simulink model "WiperSystem"  (R2016a)
settings: Solver=FixedStepDiscrete  StartTime=0.0  StopTime=20  FixedStep=0.01  RelTol=1e-3
undefined symbols (not defined in the file): sigbuilder_block
libraries: simulink x1
settings Model: Creator=Kimo Store  LastModifiedBy=Kimo Store

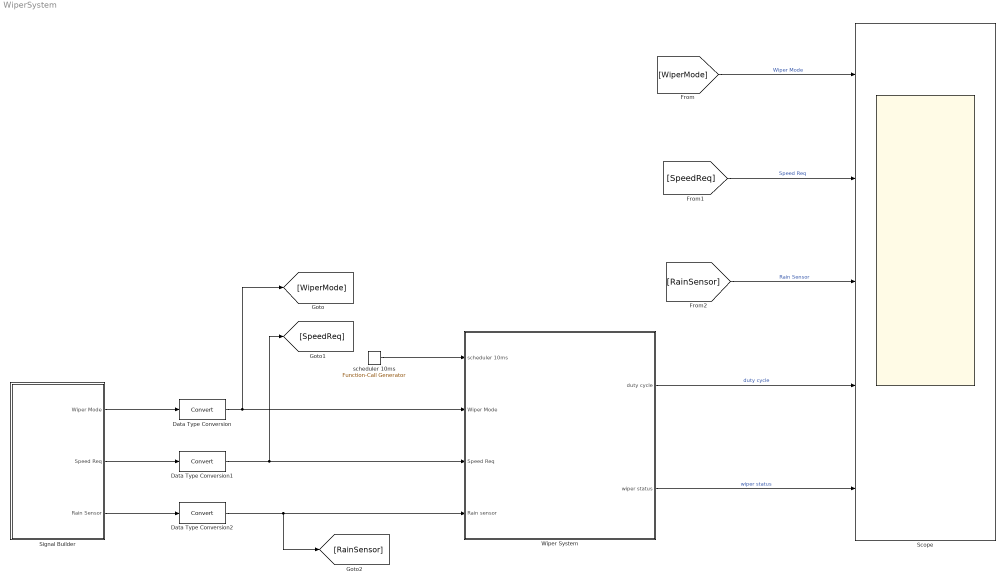
== system WiperSystem ==
  Data Type Conversion : DataTypeConversion
  Data Type Conversion1 : DataTypeConversion
  Data Type Conversion2 : DataTypeConversion
  Scope : Scope  NumInputPorts=5
  Signal Builder : Subsystem  Tag=STV Subsys  LoadFcn=sigbuilder_block('load');  StartFcn=sigbuilder_block('start');  StopFcn=sigbuilder_block('stop');  ClipboardFcn=sigbuilder_block('clipboard');  mask(Sigbuilder block){}
      mask help: Simulink:masks:SigbuilderBlock_MD
      mask init:
      | if ~strcmp(get_param(bdroot(gcbh),'SimulationStatus'),'stopped') tuvar = sigbuilder_block('maskInit'); end
      settings: CopyFcn=sigbuilder_block('copy');  DeleteFcn=sigbuilder_block('delete');  ModelCloseFcn=sigbuilder_block('modelClose');  PreSaveFcn=sigbuilder_block('preSave');  PauseFcn=sigbuilder_block('pause');  ContinueFcn=sigbuilder_block('continue');  NameChangeFcn=sigbuilder_block('namechange');  OpenFcn=sigbuilder_block('open',[5.4 30 1141.2 522.6 ]);  CloseFcn=sigbuilder_block('close');
      mask Display: plot(0, 0, 100, 100,[2, 2, 32, 32, 2], [68, 8, 8, 68, 68],[32, 2], [38, 38], [32, 19, 2],[53, 60, 44], [32, 17, 17, 2],[16, 16, 31, 31]);txt = getActiveGroup(gcbh);text(2, 100, txt,'verticalAlignment', 'top');
  Wiper System : Subsystem
  scheduler 10ms : simulink/Ports & Subsystems/Function-Call Generator  sample_time=0.01  numberOfIterations=1
  wires:
  scheduler 10ms/1 -> Wiper System/1(scheduler 10ms)
  Wiper System/2(wiper status) -> Scope/5  "wiper status"
  Wiper System/1(duty cycle) -> Scope/4  "duty cycle"
  Signal Builder/1(Wiper Mode) -> Data Type Conversion/1
  Data Type Conversion/1 -> [WiperMode], Wiper System/2(Wiper Mode)
  Data Type Conversion1/1 -> [SpeedReq], Wiper System/3(Speed Req)
  Data Type Conversion2/1 -> [RainSensor], Wiper System/4(Rain sensor)
  [WiperMode] -> Scope/1  "Wiper Mode"
  [SpeedReq] -> Scope/2  "Speed Req"
  [RainSensor] -> Scope/3  "Rain Sensor"
  Signal Builder/2(Speed Req) -> Data Type Conversion1/1
  Signal Builder/3(Rain Sensor) -> Data Type Conversion2/1

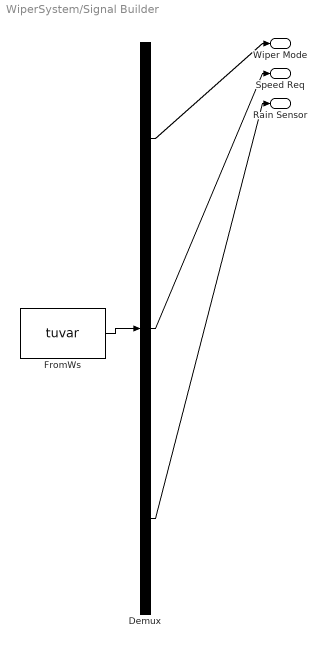
== system WiperSystem/Signal Builder ==
  Demux : Demux  Tag=STV Demux  Outputs=3
  FromWs : FromWorkspace  Tag=STV FromWs  VariableName=tuvar  SampleTime=0
      SigBuilderData=|
      | common.afterFinalStr = 'Extrapolate'
      | common.sampleTime = 0
      | dataSet.timeRange = [0 20]
      | dataSet.name = 'Group 1'
      | sbobj.Groups.Name = 'Group 1'
      | sbobj.Groups.Signals(1).Name = 'Wiper Mode'
      | sbobj.Groups.Signals(1).XData = [0 1 2 3 4 5 6 20]
      | sbobj.Groups.Signals(1).YData = [0 0 2 2 3 3 1 1]
      | sbobj.Groups.Signals(2).Name = 'Speed Req'
      | sbobj.Groups.Signals(2).XData = [0 7 8 9 10 11 12 13 14 20]
      | sbobj.Groups.Signals(2).YData = [0 0 1 2 3 4 5 6 7 7]
      | sbobj.Groups.Signals(3).Name = 'Rain Sensor'
      | sbobj.Groups.Signals(3).XData = [0 14 15 15.56 16 20]
      | sbobj.Groups.Signals(3).YData = [0 0 1 0.44 0 0]
      | sbobj.Groups.TimeRange = [0 20]
  Wiper Mode : Outport  Tag=STV Outport
  Speed Req : Outport  Tag=STV Outport  Port=2
  Rain Sensor : Outport  Tag=STV Outport  Port=3
  wires:
  FromWs/1 -> Demux/1
  Demux/1 -> Wiper Mode/1
  Demux/2 -> Speed Req/1
  Demux/3 -> Rain Sensor/1

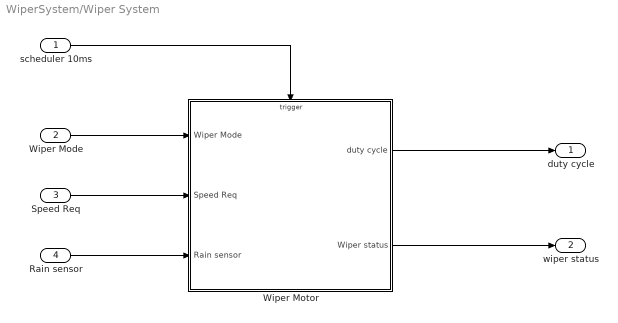
== system WiperSystem/Wiper System ==
  scheduler 10ms : Inport
  Wiper Mode : Inport  Port=2  OutDataTypeStr=uint8
  Speed Req : Inport  Port=3  OutDataTypeStr=uint8
  Rain sensor : Inport  Port=4  OutDataTypeStr=boolean
  Wiper Motor : Subsystem  TreatAsAtomicUnit=on
  duty cycle : Outport  OutDataTypeStr=single
  wiper status : Outport  Port=2  OutDataTypeStr=boolean
  wires:
  Wiper Motor/1(duty cycle) -> duty cycle/1
  Speed Req/1 -> Wiper Motor/2(Speed Req)
  Rain sensor/1 -> Wiper Motor/3(Rain sensor)
  Wiper Motor/2(Wiper status) -> wiper status/1
  scheduler 10ms/1 -> Wiper Motor/Trigger
  Wiper Mode/1 -> Wiper Motor/1(Wiper Mode)

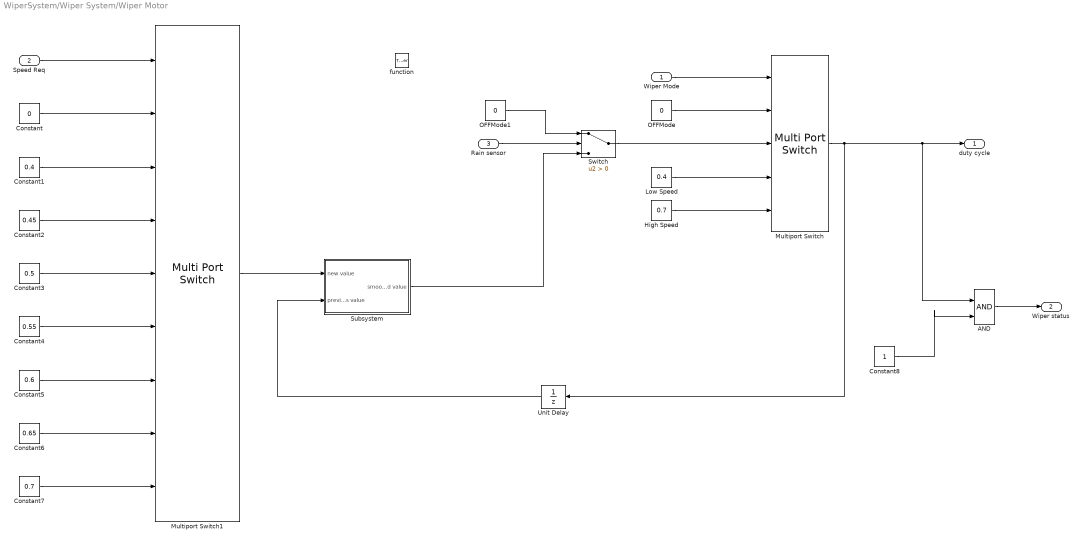
== system WiperSystem/Wiper System/Wiper Motor ==
  Wiper Mode : Inport
  Speed Req : Inport  Port=2  OutDataTypeStr=uint8
  Rain sensor : Inport  Port=3
  function : TriggerPort  TriggerType=function-call  VariantControl=Variant
  AND : Logic  IconShape=distinctive  AllPortsSameDT=off  OutDataTypeStr=boolean
  Constant : Constant  Value=0
  Constant1 : Constant  Value=0.4
  Constant2 : Constant  Value=0.45
  Constant3 : Constant  Value=0.5
  Constant4 : Constant  Value=0.55
  Constant5 : Constant  Value=0.6
  Constant6 : Constant  Value=0.65
  Constant7 : Constant  Value=0.7
  Constant8 : Constant
  High Speed : Constant  Value=0.7  OutDataTypeStr=single
  Low Speed : Constant  Value=0.4  OutDataTypeStr=single
  Multiport Switch : MultiPortSwitch  DataPortOrder=Zero-based contiguous  Inputs=4
  Multiport Switch1 : MultiPortSwitch  DataPortOrder=Zero-based contiguous  Inputs=8
  OFFMode : Constant  Value=0  OutDataTypeStr=single
  OFFMode1 : Constant  Value=0
  Subsystem : Subsystem
  Switch : Switch  Criteria=u2 > Threshold  OutDataTypeStr=single
  Unit Delay : UnitDelay  SampleTime=-1
  duty cycle : Outport
  Wiper status : Outport  Port=2
  wires:
  Wiper Mode/1 -> Multiport Switch/1
  OFFMode/1 -> Multiport Switch/2
  High Speed/1 -> Multiport Switch/5
  Low Speed/1 -> Multiport Switch/4
  Switch/1 -> Multiport Switch/3
  OFFMode1/1 -> Switch/1
  Rain sensor/1 -> Switch/2
  Speed Req/1 -> Multiport Switch1/1
  Constant/1 -> Multiport Switch1/2
  Constant2/1 -> Multiport Switch1/4
  Constant3/1 -> Multiport Switch1/5
  Constant4/1 -> Multiport Switch1/6
  Constant5/1 -> Multiport Switch1/7
  Constant6/1 -> Multiport Switch1/8
  Constant7/1 -> Multiport Switch1/9
  Multiport Switch1/1 -> Subsystem/1(new value)
  Subsystem/1(smoothed value) -> Switch/3
  Multiport Switch/1 -> Unit Delay/1, AND/1, duty cycle/1
  AND/1 -> Wiper status/1
  Constant8/1 -> AND/2
  Unit Delay/1 -> Subsystem/2(previous value)
  Constant1/1 -> Multiport Switch1/3

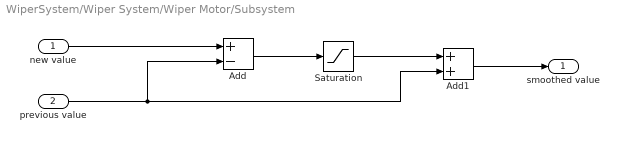
== system WiperSystem/Wiper System/Wiper Motor/Subsystem ==
  new value : Inport
  previous value : Inport  Port=2
  Add : Sum  Inputs=+-
  Add1 : Sum
  Saturation : Saturate  UpperLimit=0.005
  smoothed value : Outport
  wires:
  new value/1 -> Add/1
  previous value/1 -> Add/2, Add1/2
  Add/1 -> Saturation/1
  Saturation/1 -> Add1/1
  Add1/1 -> smoothed value/1
